simulink model "Kalmanfilter"  (R2016a)
settings: Solver=VariableStepAuto  StartTime=0.0  StopTime=10.0  RelTol=1e-3
settings Model: Creator=24535  LastModifiedBy=24535

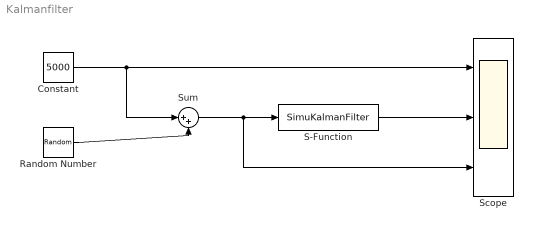
== system Kalmanfilter ==
  Constant : Constant  Value=5000
  Random Number : RandomNumber  Variance=5  SampleTime=0.1
  S-Function : S-Function  FunctionName=SimuKalmanFilter  SFunctionDeploymentMode=off  EnableBusSupport=off
  Scope : Scope  NumInputPorts=3
  Sum : Sum  Inputs=|++
  wires:
  Constant/1 -> Scope/1, Sum/1
  Random Number/1 -> Sum/2
  Sum/1 -> Scope/3, S-Function/1
  S-Function/1 -> Scope/2
